simulink model "malicious_pilot"  (Simulink 4.00)
settings: Solver=ode45  StartTime=0.0  StopTime=4*pi  MaxStep=0.001*pi  RelTol=1e-3
settings Model: LastModifiedBy=acataldo

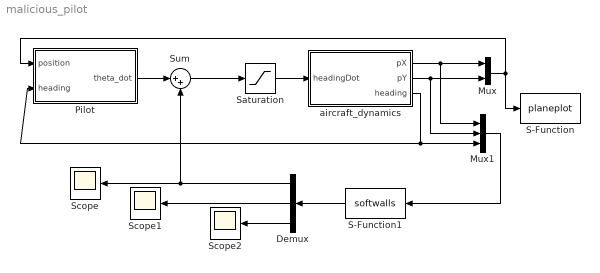
== system malicious_pilot ==
  Demux : Demux  Orientation=left  Outputs=3  BusSelectionMode=off
  Mux : Mux  Inputs=2
  Mux1 : Mux  Inputs=3
  Pilot : Subsystem
      settings: RTWFcnNameOpts=Auto  RTWFileNameOpts=Auto
  S-Function : S-Function  FunctionName=planeplot  PortCounts=[]  SFunctionModules=''
  S-Function1 : S-Function  Orientation=left  FunctionName=softwalls  PortCounts=[]  SFunctionModules=''
  Saturation : Saturate  UpperLimit=1.0 / 0.15  LowerLimit=-1.0 / 0.15  LinearizeAsGain=on
  Scope : Scope
      settings: TimeRange=auto  YMin=-250  YMax=300  SaveToWorkspace=off  SaveName=ScopeData  LimitDataPoints=on  MaxDataPoints=5000
  Scope1 : Scope
      settings: TimeRange=auto  YMin=-5  YMax=5  SaveToWorkspace=off  LimitDataPoints=on  MaxDataPoints=5000
  Scope2 : Scope
      settings: TimeRange=auto  YMin=-5  YMax=5  SaveToWorkspace=off  SaveName=ScopeData2  LimitDataPoints=on  MaxDataPoints=5000
  Sum : Sum  Inputs=|++  SaturateOnIntegerOverflow=on
  aircraft_dynamics : Subsystem  TreatAsAtomicUnit=on
      settings: RTWFcnNameOpts=Auto  RTWFileNameOpts=Auto
  wires:
  Pilot/1(theta_dot) -> Sum/1
  aircraft_dynamics/1(pX) -> Mux/1, Mux1/1
  aircraft_dynamics/2(pY) -> Mux/2, Mux1/2
  Mux/1 -> S-Function/1, Pilot/1(position)
  aircraft_dynamics/3(heading) -> Mux1/3, Pilot/2(heading)
  Mux1/1 -> S-Function1/1
  Sum/1 -> Saturation/1
  Saturation/1 -> aircraft_dynamics/1(headingDot)
  S-Function1/1 -> Demux/1
  Demux/1 -> Scope/1, Sum/2
  Demux/2 -> Scope1/1
  Demux/3 -> Scope2/1

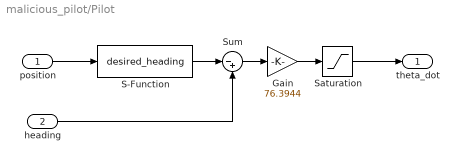
== system malicious_pilot/Pilot ==
  position : Inport  Port=1  LatchInput=off
  heading : Inport  Port=2  LatchInput=off
  Gain : Gain  Gain=76.3944  Multiplication=Element-wise(K.*u)  SaturateOnIntegerOverflow=on
  S-Function : S-Function  FunctionName=desired_heading  PortCounts=[]  SFunctionModules=''
  Saturation : Saturate  UpperLimit=1 / 0.15  LowerLimit=-1 / 0.15  LinearizeAsGain=on
  Sum : Sum  Inputs=|-+  SaturateOnIntegerOverflow=on
  theta_dot : Outport  Port=1
  wires:
  position/1 -> S-Function/1
  S-Function/1 -> Sum/1
  heading/1 -> Sum/2
  Sum/1 -> Gain/1
  Gain/1 -> Saturation/1
  Saturation/1 -> theta_dot/1

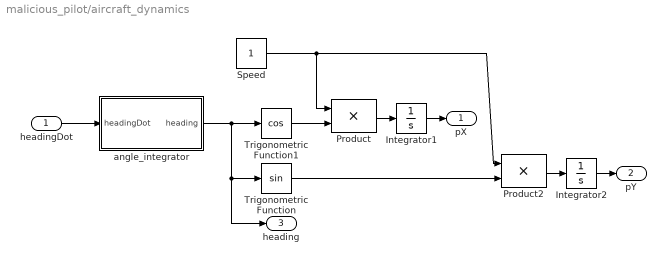
== system malicious_pilot/aircraft_dynamics ==
  headingDot : Inport  Port=1  LatchInput=off
  Integrator1 : Integrator  ExternalReset=none  InitialConditionSource=internal  InitialCondition=0  LimitOutput=off  UpperSaturationLimit=inf  LowerSaturationLimit=-inf  ShowSaturationPort=off  ShowStatePort=off  AbsoluteTolerance=auto
  Integrator2 : Integrator  ExternalReset=none  InitialConditionSource=internal  InitialCondition=0  LimitOutput=off  UpperSaturationLimit=inf  LowerSaturationLimit=-inf  ShowSaturationPort=off  ShowStatePort=off  AbsoluteTolerance=auto
  Product : Product  Inputs=2  Multiplication=Element-wise(.*)  SaturateOnIntegerOverflow=on
  Product2 : Product  Inputs=2  Multiplication=Element-wise(.*)  SaturateOnIntegerOverflow=on
  Speed : Constant  Value=1
  Trigonometric Function : Trigonometry  Operator=sin  OutputSignalType=auto
  Trigonometric Function1 : Trigonometry  Operator=cos  OutputSignalType=auto
  angle_integrator : Subsystem  TreatAsAtomicUnit=on
      settings: RTWFcnNameOpts=Auto  RTWFileNameOpts=Auto
  pX : Outport  Port=1
  pY : Outport  Port=2
  heading : Outport  Port=3
  wires:
  Speed/1 -> Product/1, Product2/1
  angle_integrator/1(heading) -> Trigonometric Function1/1, Trigonometric Function/1, heading/1
  Trigonometric Function1/1 -> Product/2
  Trigonometric Function/1 -> Product2/2
  Product/1 -> Integrator1/1
  Integrator1/1 -> pX/1
  Product2/1 -> Integrator2/1
  Integrator2/1 -> pY/1
  headingDot/1 -> angle_integrator/1(headingDot)

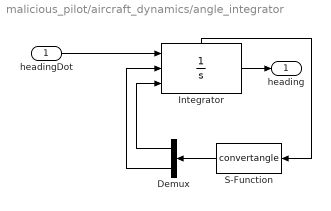
== system malicious_pilot/aircraft_dynamics/angle_integrator ==
  headingDot : Inport  Port=1  LatchInput=off
  Demux : Demux  Orientation=left  Outputs=2  BusSelectionMode=off
  Integrator : Integrator  ExternalReset=level  InitialConditionSource=external  InitialCondition=0  LimitOutput=off  UpperSaturationLimit=inf  LowerSaturationLimit=-inf  ShowSaturationPort=off  ShowStatePort=on  AbsoluteTolerance=auto
  S-Function : S-Function  Orientation=left  FunctionName=convertangle  PortCounts=[]  SFunctionModules=''
  heading : Outport  Port=1
  wires:
  headingDot/1 -> Integrator/1
  Integrator/1 -> heading/1
  S-Function/1 -> Demux/1
  Demux/1 -> Integrator/3
  Demux/2 -> Integrator/2
  Integrator/State -> S-Function/1
